simulink library "Differential_Gear1DShafts1D"  (R2026a)
settings: Solver=VariableStepAuto
libraries: fl_lib x2, nesl_utility x2, sdl_lib x1, sm_lib x1
Description:
  | Component of Simscape Vehicle Templates Library
  | 
  | Copyright 2018-2026 The MathWorks, Inc.
settings Model: Creator=smiller  LastModifiedBy=smiller

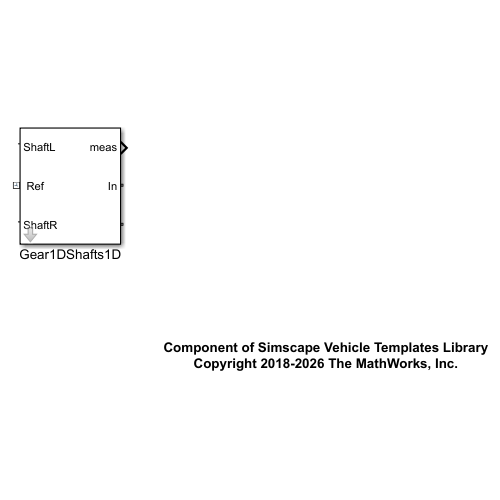
[thumbnail: Simulink's stored preview of the top-level diagram]
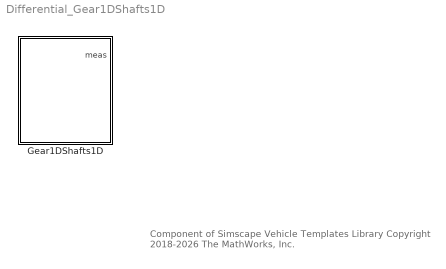
== system Differential_Gear1DShafts1D ==
  note: Component of Simscape Vehicle Templates Library
      | Copyright 2018-2026 The MathWorks, Inc.
  Gear1DShafts1D : Subsystem  VariantControl=Gear1DShafts1D  mask(Differential with 1D shafts){}
      mask help: Models differential with 1D mechanical shafts.

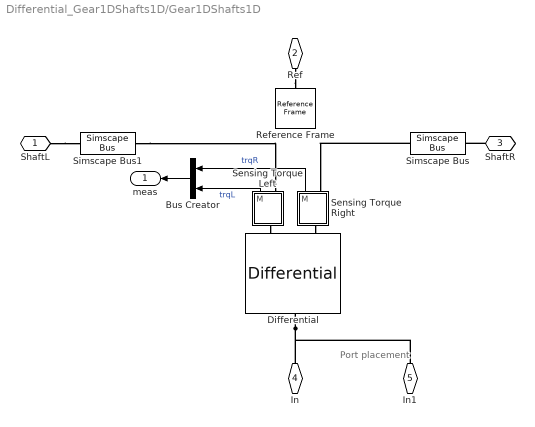
== system Differential_Gear1DShafts1D/Gear1DShafts1D ==
  note: Port
      | placement
  Bus Creator : BusCreator  Inputs=2
  Differential : sdl_lib/Gears/Differential  driveshaft_location=2  cd_ratio=Differential.ratio.Value  friction_model=1  efficiency=[.85, .92]  temperature_TLU=[280, 300, 320] K  efficiency_ss_TLU=[.95, .9, .85]  efficiency_cd_TLU=[.95, .9, .85]  pwr_thr=[.001, .001] W  mu_visc=[0, 0] N*m/(rad/s)  model_inertia=0  sun_inertia=1e-10 kg*m^2  sun_radius=0.01 m  carrier_inertia=0.001 kg*m^2  planet_inertia=0.001 kg*m^2  planet_mass=1e-10 kg  thermal_mass=50 J/K  T_init=300 K
  Reference Frame : sm_lib/Frames and Transforms/Reference Frame
  Sensing Torque Left : Subsystem
  Sensing Torque Right : Subsystem
  Simscape Bus : SimscapeBus  HierarchyStrings=Shaft1D
  Simscape Bus1 : SimscapeBus  HierarchyStrings=Shaft1D
  ShaftL : PMIOPort  Side=Left
  " Ref" : PMIOPort  Port=2  Side=Left
  ShaftR : PMIOPort  Port=3  Side=Left
  In : PMIOPort  Port=4  Side=Right
  In1 : PMIOPort  Port=5  Side=Right
  meas : Outport  VectorParamsAs1DForOutWhenUnconnected=off
  wires:
  Sensing Torque Right/1(M) -> Bus Creator/1  "trqR"
  Sensing Torque Left/1(M) -> Bus Creator/2  "trqL"
  Bus Creator/1 -> meas/1
  connections:
  Sensing Torque Right/LConn1 -- Differential/RConn1
  Sensing Torque Left/LConn1 -- Differential/RConn2
  ShaftL/RConn1 -- Simscape Bus1/RConn1
  ShaftR/RConn1 -- Simscape Bus/RConn1
  Simscape Bus1/LConn1 -- Sensing Torque Left/RConn1
  " Ref"/RConn1 -- Reference Frame/RConn1
  Simscape Bus/LConn1 -- Sensing Torque Right/RConn1
  Differential/LConn1 -- In1/RConn1 -- In/RConn1

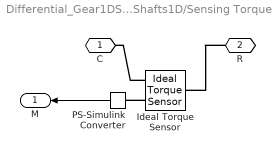
== system Differential_Gear1DShafts1D/Gear1DShafts1D/Sensing Torque Left ==
  Ideal Torque Sensor : fl_lib/Mechanical/Mechanical Sensors/Ideal Torque Sensor
  PS-Simulink Converter : nesl_utility/PS-Simulink Converter  PhysicalDomain=network_engine_domain  SubClassName=ps_output  LeftPortType=input  RightPortType=output  PseudoPeriodic=off  Frequencies=[]  VectorFormat=1-D array  Unit=N*m  AffineConversion=off
  C : PMIOPort  Side=Right
  R : PMIOPort  Port=2  Side=Left
  M : Outport  VectorParamsAs1DForOutWhenUnconnected=off
  wires:
  PS-Simulink Converter/1 -> M/1
  connections:
  Ideal Torque Sensor/RConn2 -- PS-Simulink Converter/LConn1
  R/RConn1 -- Ideal Torque Sensor/LConn1
  Ideal Torque Sensor/RConn1 -- C/RConn1

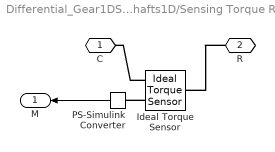
== system Differential_Gear1DShafts1D/Gear1DShafts1D/Sensing Torque Right ==
  Ideal Torque Sensor : fl_lib/Mechanical/Mechanical Sensors/Ideal Torque Sensor
  PS-Simulink Converter : nesl_utility/PS-Simulink Converter  PhysicalDomain=network_engine_domain  SubClassName=ps_output  LeftPortType=input  RightPortType=output  PseudoPeriodic=off  Frequencies=[]  VectorFormat=1-D array  Unit=N*m  AffineConversion=off
  C : PMIOPort  Side=Right
  R : PMIOPort  Port=2  Side=Left
  M : Outport  VectorParamsAs1DForOutWhenUnconnected=off
  wires:
  PS-Simulink Converter/1 -> M/1
  connections:
  Ideal Torque Sensor/RConn1 -- C/RConn1
  R/RConn1 -- Ideal Torque Sensor/LConn1
  Ideal Torque Sensor/RConn2 -- PS-Simulink Converter/LConn1
